simulink model "lab5"  (Simulink 10.0)
settings: Solver=ode23  StartTime=0.0  StopTime=5  RelTol=1e-3  EnableMultiTasking=on
InitFcn:
  | lab5i
values from neighbouring files (symbols this model uses):
  Ax = 0.03    [lab5i.m]
  Ay = 0.03    [lab5i.m]
  Az = 0    [lab5i.m]
  Kd = diag(Kd)    [lab5i.m]
  Kp = diag(Kp)    [lab5i.m]
  w0 = pi/4    (= 0.785398163397)    [lab5i.m]
  x0 = 0.15    [lab5i.m]
  y0 = 0    [lab5i.m]
  z0 = 0.035    [lab5i.m]
libraries: ELE819m x2
settings Model: Creator=Admin  LastModifiedBy=nicholasprayogo
settings DataIOCC: LimitDataPoints=on  SignalLoggingSaveFormat=ModelDataLogs
settings OptimizationCC: ExpressionDepthLimit=2147483647
settings DebuggingCC: AlgebraicLoopMsg=none  FcnCallInpInsideContextMsg=warning  StateNameClashWarn=warning
settings SFSimCC: SimParseCustomCode=off
settings GRTTargetCC: GeneratePreprocessorConditionals=Disable all
settings ConfigComp: CovExternalEMLEnable=off

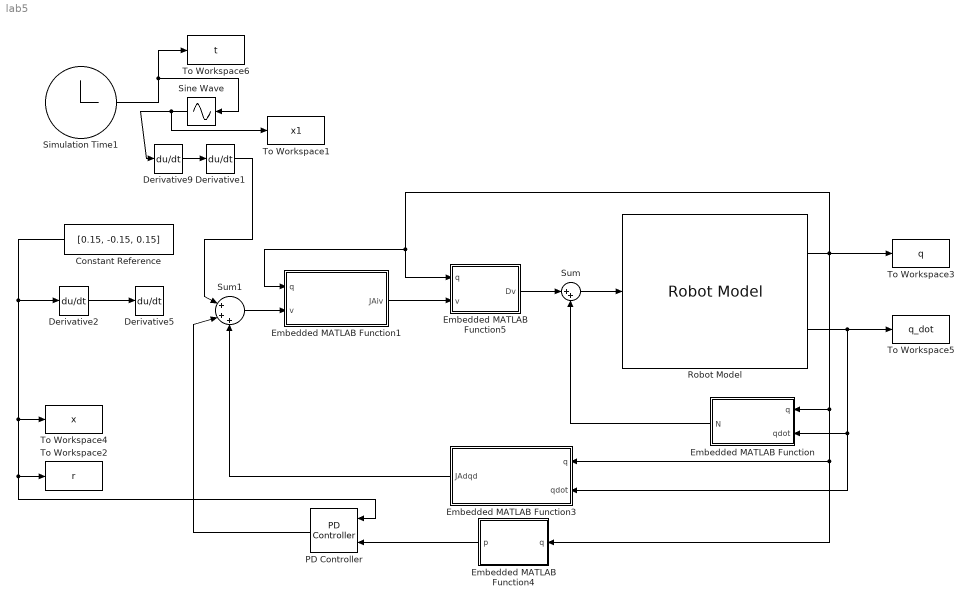
== system lab5 ==
  Constant Reference : Constant  Value=[0.15, -0.15, 0.15]
  Derivative{1..2,5,9} (4 alike) : Derivative  CoefficientInTFapproximation=0
  Embedded MATLAB Function : MATLAB Function  TreatAsAtomicUnit=on
  Embedded MATLAB Function1 : MATLAB Function  TreatAsAtomicUnit=on
  Embedded MATLAB Function3 : MATLAB Function  TreatAsAtomicUnit=on
  Embedded MATLAB Function4 : MATLAB Function  TreatAsAtomicUnit=on
  Embedded MATLAB Function5 : MATLAB Function  TreatAsAtomicUnit=on
  PD Controller : ELE819m/PD Controller  P=Kp  D=Kd  wp=wp  wd=wd
  Robot Model : ELE819m/Robot Model  q1_0=q1_0  q2_0=q2_0  q3_0=q3_0
  Simulation Time1 : Clock
      settings: Decimation=200
  Sine Wave : Sin  TimeSource=Use external signal  Amplitude="[Ax, Ay,  Az]"  Bias=[x0, y0, z0]  Frequency=[w0, w0, w0]  Phase=[0.0, pi/2, 0.0]
  Sum : Sum  Inputs=|++
  Sum1 : Sum  Inputs=|+++
  To Workspace1 : ToWorkspace  VariableName=x1  SampleTime=-1
  To Workspace2 : ToWorkspace  VariableName=r  SampleTime=-1
  To Workspace3 : ToWorkspace  VariableName=q  SampleTime=-1
      settings: Decimation=200
  To Workspace4 : ToWorkspace  VariableName=x  SampleTime=-1
  To Workspace5 : ToWorkspace  VariableName=q_dot  SampleTime=-1
      settings: Decimation=200
  To Workspace6 : ToWorkspace  VariableName=t  SampleTime=-1
      settings: Decimation=200
  wires:
  Embedded MATLAB Function4/1(p) -> PD Controller/2
  Robot Model/1 -> To Workspace3/1, Embedded MATLAB Function4/1(q), Embedded MATLAB Function3/1(q), Embedded MATLAB Function/1(q), Embedded MATLAB Function5/1(q), Embedded MATLAB Function1/1(q)
  Robot Model/2 -> To Workspace5/1, Embedded MATLAB Function3/2(qdot), Embedded MATLAB Function/2(qdot)
  Embedded MATLAB Function/1(N) -> Sum/2
  Sum/1 -> Robot Model/1
  Embedded MATLAB Function5/1(Dv) -> Sum/1
  Embedded MATLAB Function1/1(JAiv) -> Embedded MATLAB Function5/2(v)
  Sum1/1 -> Embedded MATLAB Function1/2(v)
  Simulation Time1/1 -> To Workspace6/1, Sine Wave/1
  Constant Reference/1 -> PD Controller/1, To Workspace2/1, To Workspace4/1, Derivative2/1
  Derivative2/1 -> Derivative5/1
  Embedded MATLAB Function3/1(JAdqd) -> Sum1/3
  PD Controller/1 -> Sum1/2
  Sine Wave/1 -> To Workspace1/1, Derivative9/1
  Derivative9/1 -> Derivative1/1
  Derivative1/1 -> Sum1/1

== matlab function Embedded MATLAB Function1 ==
  data: q input double; v input double; JAiv output double
function JAiv = JAInvV_blk(q, v)
%#eml
JAiv = JAInvV(q, v);

== matlab function Embedded MATLAB Function ==
  data: q input double; N output double; qdot input double
function N = N_blk(q, qdot)
%#eml
N = nterm(q, qdot);

== matlab function Embedded MATLAB Function3 ==
  data: q input double; JAdqd output double; qdot input double
function JAdqd = JAdotQdot_blk(q, qdot)
%#eml
JAdqd = JAdotQdot(q, qdot);

== matlab function Embedded MATLAB Function4 ==
  data: q input double; p output double
function p = for_kin_blk(q)
%#eml
p = for_kin(q);

== matlab function Embedded MATLAB Function5 ==
  data: q input double; v input double; Dv output double
function Dv = D_blk(q, v)
%#eml
Dv = dterm(q, v);
